simulink model "ACC_MP1_b"  (R2020b)
settings: Solver=ode2  StartTime=0.0  StopTime=endTime  FixedStep=Ts  RelTol=1e-3
values from neighbouring files (symbols this model uses):
  dSafe = 5    [ACCBreach_MP1_b.m]
  Ts = 0.01    [ACCBreach_MP1_b.m]
  v0_host = 0    [ACCBreach_MP1_b.m]
  vref_host = 0    [ACCBreach_MP1_b.m]
  x0_host = 0    [ACCBreach_MP1_b.m]
settings Model: Creator=jyotirmoy  LastModifiedBy=cameronakhavan
settings DataIOCC: ReturnWorkspaceOutputs=off
settings DebuggingCC: ArithmeticOperatorsInVariantConditions=warning
settings SFSimCC: SimUseLocalCustomCode=off  CustomCodeUndefinedFunction=UseInterfaceOnly
settings RTWCC: RTWUseLocalCustomCode=off
settings CodeAppCC: StateflowObjectComments=on

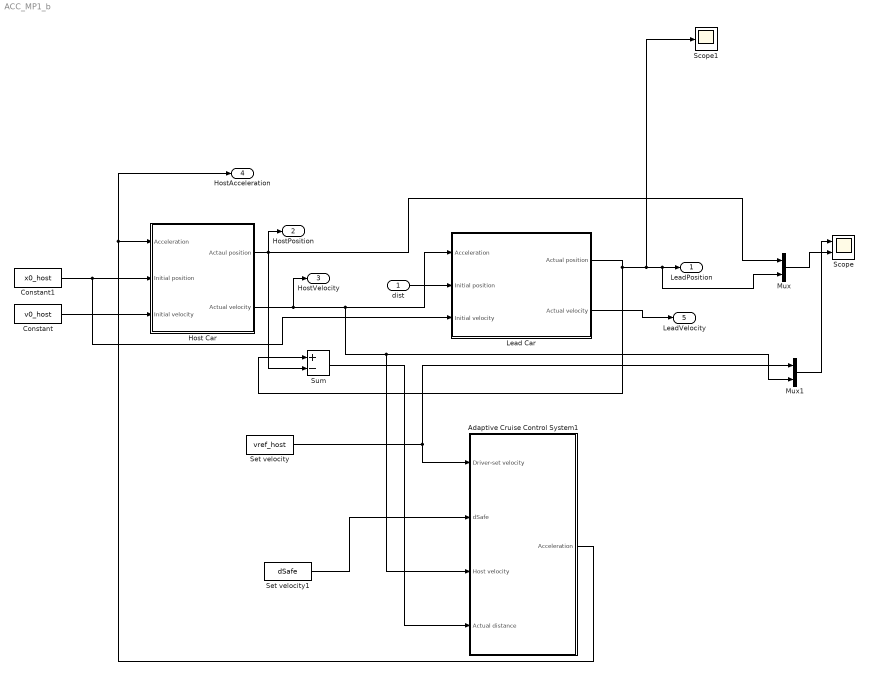
== system ACC_MP1_b ==
  dist : Inport
  Adaptive Cruise Control System1 : Subsystem  VariantControl=MODE==4
  Constant : Constant  Value=v0_host
  Constant1 : Constant  Value=x0_host
  Host Car : Subsystem
  Lead Car : Subsystem
  Mux : Mux  Inputs=2
  Mux1 : Mux  Inputs=2
  Scope : Scope  NumInputPorts=2
  Scope1 : Scope
  Set velocity : Constant  Value=vref_host  SampleTime=Ts
  Set velocity1 : Constant  Value=dSafe  SampleTime=Ts
  Sum : Sum  Inputs=+-
  LeadPosition : Outport  VectorParamsAs1DForOutWhenUnconnected=off
  HostPosition : Outport  Port=2  VectorParamsAs1DForOutWhenUnconnected=off
  HostVelocity : Outport  Port=3  VectorParamsAs1DForOutWhenUnconnected=off
  HostAcceleration : Outport  Port=4  VectorParamsAs1DForOutWhenUnconnected=off
  LeadVelocity : Outport  Port=5  VectorParamsAs1DForOutWhenUnconnected=off
  wires:
  Host Car/1(Actaul position) -> Mux/1, Sum/2, HostPosition/1
  Set velocity/1 -> Adaptive Cruise Control System1/1(Driver-set velocity), Mux1/1
  Sum/1 -> Adaptive Cruise Control System1/4(Actual distance)
  Host Car/2(Actual velocity) -> Lead Car/1(Acceleration), Adaptive Cruise Control System1/3(Host velocity), Mux1/2, HostVelocity/1
  Constant/1 -> Host Car/3(Initial velocity)
  Constant1/1 -> Lead Car/3(Initial velocity), Host Car/2(Initial position)
  Lead Car/1(Actual position) -> Scope1/1, Mux/2, LeadPosition/1, Sum/1
  Mux/1 -> Scope/2
  Mux1/1 -> Scope/1
  Lead Car/2(Actual velocity) -> LeadVelocity/1
  dist/1 -> Lead Car/2(Initial position)
  Adaptive Cruise Control System1/1("Acceleration ") -> HostAcceleration/1, Host Car/1(Acceleration)
  Set velocity1/1 -> Adaptive Cruise Control System1/2(dSafe)

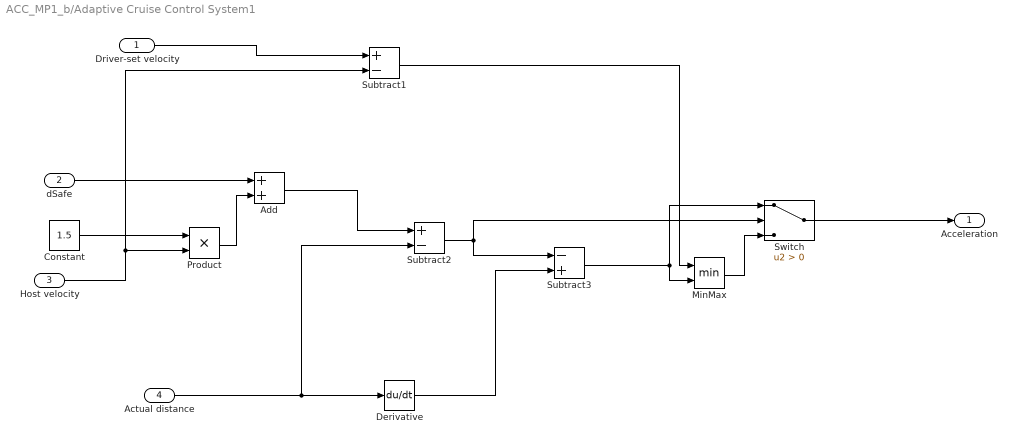
== system ACC_MP1_b/Adaptive Cruise Control System1 ==
  Driver-set velocity : Inport
  dSafe : Inport  Port=2
  Host velocity : Inport  Port=3
  Actual distance : Inport  Port=4
  Add : Sum
  Constant : Constant  Value=1.5
  Derivative : Derivative
  MinMax : MinMax  Inputs=2
  Product : Product
  Subtract1 : Sum  Inputs=+-
  Subtract2 : Sum  Inputs=+-
  Subtract3 : Sum  Inputs=-+
  Switch : Switch  Criteria=u2 > Threshold
  "Acceleration " : Outport  VectorParamsAs1DForOutWhenUnconnected=off
  wires:
  Product/1 -> Add/2
  Subtract1/1 -> MinMax/1
  dSafe/1 -> Add/1
  Subtract3/1 -> MinMax/2, Switch/1
  Add/1 -> Subtract2/1
  Constant/1 -> Product/1
  Driver-set velocity/1 -> Subtract1/1
  Host velocity/1 -> Subtract1/2, Product/2
  Subtract2/1 -> Subtract3/1, Switch/2
  Switch/1 -> "Acceleration "/1
  Actual distance/1 -> Subtract2/2, Derivative/1
  MinMax/1 -> Switch/3
  Derivative/1 -> Subtract3/2

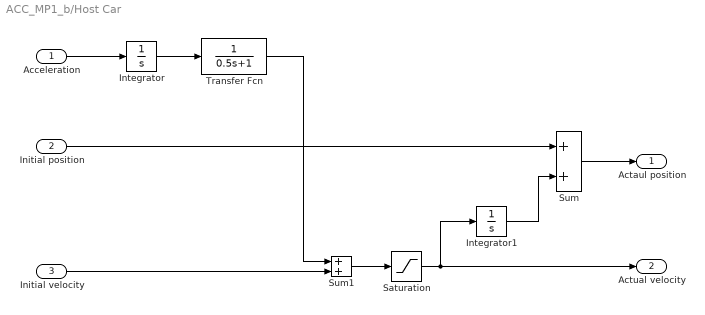
== system ACC_MP1_b/Host Car ==
  Acceleration : Inport
  Initial position : Inport  Port=2
  Initial velocity : Inport  Port=3
  Integrator : Integrator
  Integrator1 : Integrator
  Saturation : Saturate  UpperLimit=vref_host  LowerLimit=0
  Sum : Sum
  Sum1 : Sum
  Transfer Fcn : TransferFcn  Denominator=[0.5 1]
  Actaul position : Outport  VectorParamsAs1DForOutWhenUnconnected=off
  Actual velocity : Outport  Port=2  VectorParamsAs1DForOutWhenUnconnected=off
  wires:
  Initial velocity/1 -> Sum1/2
  Sum/1 -> Actaul position/1
  Transfer Fcn/1 -> Sum1/1
  Integrator/1 -> Transfer Fcn/1
  Acceleration/1 -> Integrator/1
  Initial position/1 -> Sum/1
  Integrator1/1 -> Sum/2
  Sum1/1 -> Saturation/1
  Saturation/1 -> Actual velocity/1, Integrator1/1

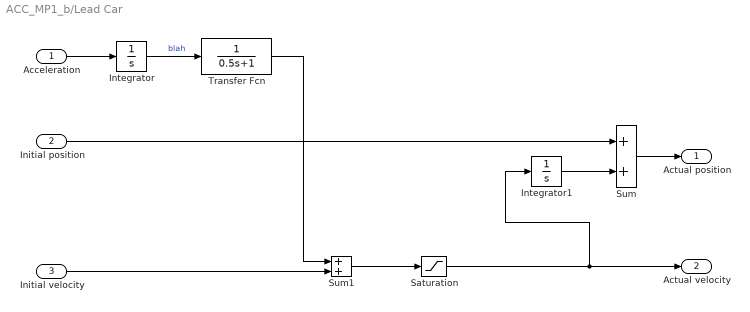
== system ACC_MP1_b/Lead Car ==
  Acceleration : Inport
  Initial position : Inport  Port=2
  Initial velocity : Inport  Port=3
  Integrator : Integrator
  Integrator1 : Integrator
  Saturation : Saturate  UpperLimit=60  LowerLimit=0
  Sum : Sum
  Sum1 : Sum
  Transfer Fcn : TransferFcn  Denominator=[0.5 1]
  Actual position : Outport  VectorParamsAs1DForOutWhenUnconnected=off
  Actual velocity : Outport  Port=2  VectorParamsAs1DForOutWhenUnconnected=off
  wires:
  Initial position/1 -> Sum/1
  Initial velocity/1 -> Sum1/2
  Integrator1/1 -> Sum/2
  Sum/1 -> Actual position/1
  Acceleration/1 -> Integrator/1
  Transfer Fcn/1 -> Sum1/1
  Sum1/1 -> Saturation/1
  Saturation/1 -> Integrator1/1, Actual velocity/1
  Integrator/1 -> Transfer Fcn/1  "blah"
